simulink model "ScanMatcher_v21"  (R2021a)
settings: Solver=FixedStepAuto  StartTime=0.0  StopTime=inf  RelTol=1e-3
model workspace (MAT data in the model file):
  SL_ROS_VariableLengthArrays_MaxSizes.CommonInfo.ArrayTruncateAction = 'EmitWarning'
  SL_ROS_VariableLengthArrays_MaxSizes.MsgTypeMap = containers.Map
  SL_ROS_VariableLengthArrays_MaxSizes.MsgTypeMap.serialization.keys = {'sensor_msgs/LaserScan'}
  SL_ROS_VariableLengthArrays_MaxSizes.MsgTypeMap.serialization.values{1}(1).PropertyName = 'Intensities'
  SL_ROS_VariableLengthArrays_MaxSizes.MsgTypeMap.serialization.values{1}(1).DataType = 'single'
  SL_ROS_VariableLengthArrays_MaxSizes.MsgTypeMap.serialization.values{1}(1).MaxLength = 1084
  SL_ROS_VariableLengthArrays_MaxSizes.MsgTypeMap.serialization.values{1}(2).PropertyName = 'Ranges'
  SL_ROS_VariableLengthArrays_MaxSizes.MsgTypeMap.serialization.values{1}(2).DataType = 'single'
  SL_ROS_VariableLengthArrays_MaxSizes.MsgTypeMap.serialization.values{1}(2).MaxLength = 1084
  SL_ROS_VariableLengthArrays_MaxSizes.MsgTypeMap.serialization.uniformity = 0
  SL_ROS_VariableLengthArrays_MaxSizes.MsgTypeMap.serialization.keyType = 'char'
  SL_ROS_VariableLengthArrays_MaxSizes.MsgTypeMap.serialization.valueType = 'any'
undefined symbols (not defined in the file): Header, Pose, Theta, X, Y
libraries: robotlib x23, robotcorelib x2
(part 1 of 2)
settings Model: Creator=roboticlab01  LastModifiedBy=roboticlab02
settings SolverCC: AlgebraicLoopSolver=TrustRegion
settings OptimizationCC: EnhancedBackFolding=on  PassReuseOutputArgsAs=Individual arguments  MaxStackSize=64  OptimizeBlockOrder=speed  DifferentSizesBufferReuse=on  OptimizationCustomize=off  EfficientTunableParamExpr=on
settings DebuggingCC: ParameterTunabilityLossMsg=error  SFMachineParentedDataDiag=warning
settings HardwareCC: ProdBitPerPointer=32  ProdBitPerSizeT=32  ProdBitPerPtrDiffT=32  ProdLargestAtomicFloat=None  ProdIntDivRoundTo=Undefined  ProdEndianess=Unspecified  ProdWordSize=32  ProdHWDeviceType=Generic->Unspecified (assume 32-bit Generic)
settings SFSimCC: MATLABDynamicMemAlloc=off  CustomCodeUndefinedFunction=UseInterfaceOnly  SimTargetLang=C++
settings RTWCC: SystemTargetFile=ert.tlc  HardwareBoard=Robot Operating System (ROS)  TLCOptions="-aInlineSetEventsForThisBaseRateFcn=TLC_FALSE -aSuppressMultiTaskScheduler=TLC_FALSE  -aRateBasedStepFcn=0"  TemplateMakefile=ert_default_tmf  GenerateReport=on  Toolchain=Catkin  IncludeHyperlinkInReport=on  LaunchReport=on  TargetLang=C++  GenerateTraceInfo=on  GenerateTraceReport=on  GenerateTraceReportSl=on  GenerateTraceReportSf=on  GenerateTraceReportEml=on
settings CodeAppCC: ForceParamTrailComments=on  IgnoreCustomStorageClasses=off  OperatorAnnotations=on  SimulinkDataObjDesc=on  SFDataObjDesc=on  InsertBlockDesc=on
settings ERTTargetCC: SupportVariableSizeSignals=on

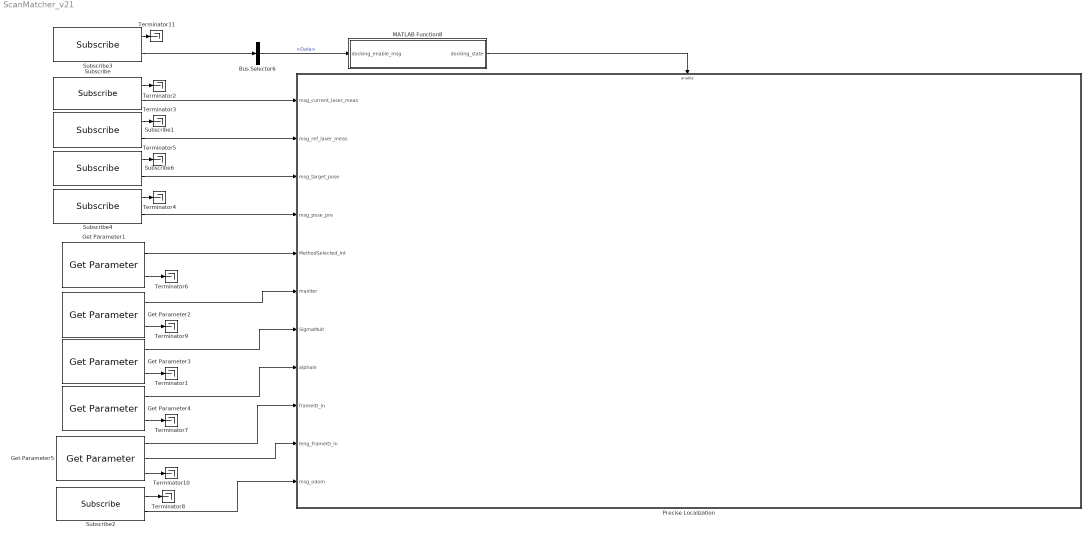
== system ScanMatcher_v21 ==
  Bus Selector6 : BusSelector  OutputSignals=Data
  Get Parameter1 : robotlib/Get Parameter  ParameterSource=Select from ROS network  ParameterName=/use_which_matcher  ParameterType=int32  ParameterMaxArrayLength=16  ParameterInitialValue=0  SampleTime=-1  ShowErrorCodeOutput=on  ModelName=ScanMatcher_v21  BlockId=ParamGet_ScanMatcher_v21_196
      settings: SourceProductBaseCode=RR
  Get Parameter2 : robotlib/Get Parameter  ParameterSource=Select from ROS network  ParameterName=/maxIter  ParameterType=int32  ParameterMaxArrayLength=16  ParameterInitialValue=100  SampleTime=-1  ShowErrorCodeOutput=on  ModelName=ScanMatcher_v21  BlockId=ParamGet_ScanMatcher_v21_325
      settings: SourceProductBaseCode=RR
  Get Parameter3 : robotlib/Get Parameter  ParameterSource=Select from ROS network  ParameterName=/sigmaMult  ParameterType=double  ParameterMaxArrayLength=16  ParameterInitialValue=1  SampleTime=-1  ShowErrorCodeOutput=on  ModelName=ScanMatcher_v21  BlockId=ParamGet_ScanMatcher_v21_340
      settings: SourceProductBaseCode=RR
  Get Parameter4 : robotlib/Get Parameter  ParameterSource=Select from ROS network  ParameterName=/alphaIn  ParameterType=double  ParameterMaxArrayLength=16  ParameterInitialValue=0.8  SampleTime=-1  ShowErrorCodeOutput=on  ModelName=ScanMatcher_v21  BlockId=ParamGet_ScanMatcher_v21_351
      settings: SourceProductBaseCode=RR
  Get Parameter5 : robotlib/Get Parameter  ParameterSource=Select from ROS network  ParameterName=/pose_frameID  ParameterType=uint8[] (string)  ParameterMaxArrayLength=32  ParameterInitialValue=0  SampleTime=-1  ShowErrorCodeOutput=on  ModelName=ScanMatcher_v21  BlockId=ParamGet_ScanMatcher_v21_466
      settings: SourceProductBaseCode=RR
  MATLAB Function8 : MATLAB Function  TreatAsAtomicUnit=on
  Precise Localization : Subsystem
  Subscribe : robotlib/Subscribe  topicSource=Select from ROS network  topic=/laser_all  messageType=sensor_msgs/LaserScan  SampleTime=-1  legacyBusStruct=off  messageQueueLength=1
  Subscribe1 : robotlib/Subscribe  topicSource=Specify your own  topic=/laser_all_ref  messageType=sensor_msgs/LaserScan  SampleTime=-1  legacyBusStruct=off  messageQueueLength=1
  Subscribe2 : robotlib/Subscribe  topicSource=Select from ROS network  topic=/odom  messageType=nav_msgs/Odometry  SampleTime=-1  legacyBusStruct=off  messageQueueLength=1
  Subscribe3 : robotlib/Subscribe  topicSource=Select from ROS network  topic=/enable_docking  messageType=std_msgs/Bool  SampleTime=-1  legacyBusStruct=off  messageQueueLength=2
      settings: SourceProductBaseCode=RO
  Subscribe4 : robotlib/Subscribe  topicSource=Specify your own  topic=/pose_estim_pre  messageType=geometry_msgs/PoseWithCovarianceStamped  SampleTime=-1  legacyBusStruct=off  messageQueueLength=1
      settings: SourceProductBaseCode=RO
  Subscribe6 : robotlib/Subscribe  topicSource=Select from ROS network  topic=/target_pose  messageType=geometry_msgs/Pose2D  SampleTime=-1  legacyBusStruct=off  messageQueueLength=1
      settings: SourceProductBaseCode=RO
  Terminator{1..11} (11 alike) : Terminator
  wires:
  Subscribe/1 -> Terminator2/1
  Subscribe1/1 -> Terminator3/1
  Subscribe4/1 -> Terminator4/1
  Subscribe6/1 -> Terminator5/1
  Get Parameter1/2 -> Terminator6/1
  Get Parameter2/2 -> Terminator9/1
  Get Parameter3/2 -> Terminator1/1
  Get Parameter4/2 -> Terminator7/1
  Subscribe2/1 -> Terminator8/1
  Get Parameter5/3 -> Terminator10/1
  Subscribe/2 -> Precise Localization/1(msg_current_laser_meas)
  Subscribe1/2 -> Precise Localization/2(msg_ref_laser_meas)
  Subscribe6/2 -> Precise Localization/3(msg_target_pose)
  Subscribe4/2 -> Precise Localization/4(msg_pose_pre)
  Get Parameter1/1 -> Precise Localization/5(MethodSelected_Int)
  Get Parameter2/1 -> Precise Localization/6(maxIter)
  Get Parameter3/1 -> Precise Localization/7(SigmaMult)
  Get Parameter4/1 -> Precise Localization/8(alphaIn)
  Get Parameter5/1 -> Precise Localization/9(frameID_in)
  Get Parameter5/2 -> Precise Localization/10(leng_frameID_in)
  Subscribe2/2 -> Precise Localization/11(msg_odom)
  Subscribe3/1 -> Terminator11/1
  MATLAB Function8/1(docking_state) -> Precise Localization/Enable
  Subscribe3/2 -> Bus Selector6/1
  Bus Selector6/1 -> MATLAB Function8/1(docking_enable_msg)  "<Data>"

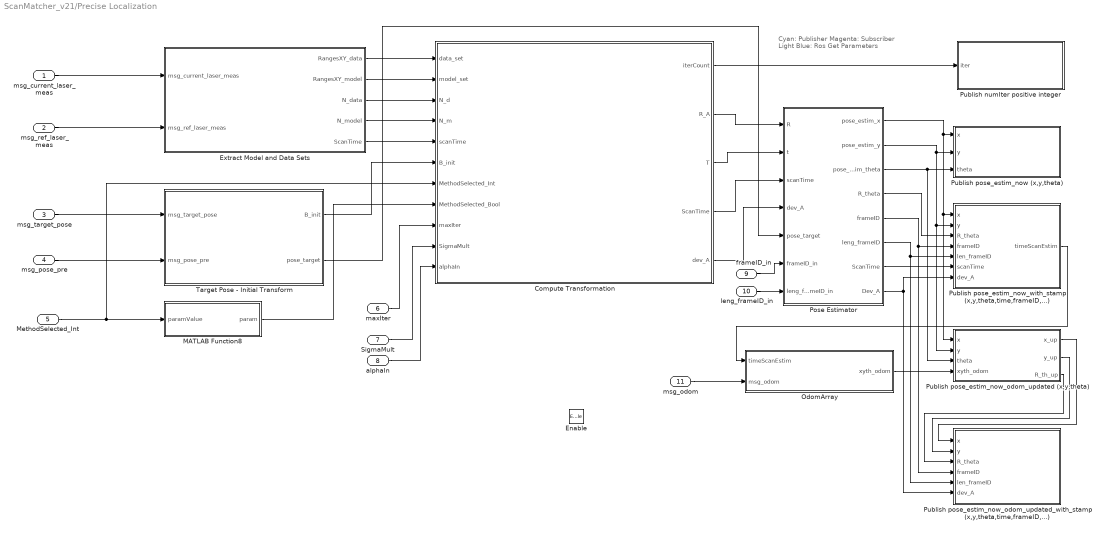
== system ScanMatcher_v21/Precise Localization ==
  note: Cyan: Publisher
      | Magenta: Subscriber
      | Light Blue: Ros Get Parameters
  msg_current_laser_meas : Inport
  msg_ref_laser_meas : Inport  Port=2
  msg_target_pose : Inport  Port=3
  msg_pose_pre : Inport  Port=4
  MethodSelected_Int : Inport  Port=5
  maxIter : Inport  Port=6
  SigmaMult : Inport  Port=7
  alphaIn : Inport  Port=8
  frameID_in : Inport  Port=9
  leng_frameID_in : Inport  Port=10
  msg_odom : Inport  Port=11
  Enable : EnablePort  PropagateVarSize=During execution
  Compute Transformation : Subsystem
  Extract Model and Data Sets : Subsystem
  MATLAB Function8 : MATLAB Function  TreatAsAtomicUnit=on
  OdomArray : Subsystem
  Pose Estimator : MATLAB Function  TreatAsAtomicUnit=on
  Publish numIter positive integer : Subsystem
  Publish pose_estim_now (x,y,theta) : Subsystem
  Publish pose_estim_now_odom_updated (x,y,theta) : Subsystem
  Publish pose_estim_now_odom_updated_with_stamp (x,y,theta,time,frameID,...) : Subsystem
  Publish pose_estim_now_with_stamp (x,y,theta,time,frameID,...) : Subsystem
  Target Pose - Initial Transform : Subsystem
  wires:
  Compute Transformation/1(iterCount) -> Publish numIter positive integer/1(iter)
  Publish pose_estim_now_odom_updated (x,y,theta)/1(x_up) -> Publish pose_estim_now_odom_updated_with_stamp (x,y,theta,time,frameID,...)/1(x)
  Extract Model and Data Sets/5(ScanTime) -> Compute Transformation/5(scanTime)
  msg_pose_pre/1 -> Target Pose - Initial Transform/2(msg_pose_pre)
  Pose Estimator/8(Dev_A) -> Publish pose_estim_now_with_stamp (x,y,theta,time,frameID,...)/7(dev_A), Publish pose_estim_now_odom_updated_with_stamp (x,y,theta,time,frameID,...)/6(dev_A)
  Compute Transformation/4(ScanTime) -> Pose Estimator/3(scanTime)
  msg_ref_laser_meas/1 -> Extract Model and Data Sets/2(msg_ref_laser_meas)
  MethodSelected_Int/1 -> Compute Transformation/7(MethodSelected_Int), MATLAB Function8/1(paramValue)
  alphaIn/1 -> Compute Transformation/11(alphaIn)
  Compute Transformation/2(R_A) -> Pose Estimator/1(R)
  maxIter/1 -> Compute Transformation/9(maxIter)
  Pose Estimator/3(pose_estim_theta) -> Publish pose_estim_now (x,y,theta)/3(theta), Publish pose_estim_now_odom_updated (x,y,theta)/3(theta)
  Compute Transformation/3(T) -> Pose Estimator/2(t)
  leng_frameID_in/1 -> Pose Estimator/7(leng_frameID_in)
  MATLAB Function8/1(param) -> Compute Transformation/8(MethodSelected_Bool)
  msg_target_pose/1 -> Target Pose - Initial Transform/1(msg_target_pose)
  Pose Estimator/5(frameID) -> Publish pose_estim_now_odom_updated_with_stamp (x,y,theta,time,frameID,...)/4(frameID), Publish pose_estim_now_with_stamp (x,y,theta,time,frameID,...)/4(frameID)
  Extract Model and Data Sets/2(RangesXY_model) -> Compute Transformation/2(model_set)
  SigmaMult/1 -> Compute Transformation/10(SigmaMult)
  msg_current_laser_meas/1 -> Extract Model and Data Sets/1(msg_current_laser_meas)
  Compute Transformation/5(dev_A) -> Pose Estimator/4(dev_A)
  Target Pose - Initial Transform/1(B_init) -> Compute Transformation/6(B_init)
  Pose Estimator/2(pose_estim_y) -> Publish pose_estim_now_odom_updated (x,y,theta)/2(y), Publish pose_estim_now_with_stamp (x,y,theta,time,frameID,...)/2(y), Publish pose_estim_now (x,y,theta)/2(y)
  Pose Estimator/6(leng_frameID) -> Publish pose_estim_now_odom_updated_with_stamp (x,y,theta,time,frameID,...)/5(len_frameID), Publish pose_estim_now_with_stamp (x,y,theta,time,frameID,...)/5(len_frameID)
  Pose Estimator/1(pose_estim_x) -> Publish pose_estim_now_odom_updated (x,y,theta)/1(x), Publish pose_estim_now_with_stamp (x,y,theta,time,frameID,...)/1(x), Publish pose_estim_now (x,y,theta)/1(x)
  Publish pose_estim_now_odom_updated (x,y,theta)/3(R_th_up) -> Publish pose_estim_now_odom_updated_with_stamp (x,y,theta,time,frameID,...)/3(R_theta)
  Target Pose - Initial Transform/2(pose_target) -> Pose Estimator/5(pose_target)
  Pose Estimator/4(R_theta) -> Publish pose_estim_now_with_stamp (x,y,theta,time,frameID,...)/3(R_theta)
  frameID_in/1 -> Pose Estimator/6(frameID_in)
  Extract Model and Data Sets/1(RangesXY_data) -> Compute Transformation/1(data_set)
  Extract Model and Data Sets/3(N_data) -> Compute Transformation/3(N_d)
  Pose Estimator/7(ScanTime) -> Publish pose_estim_now_with_stamp (x,y,theta,time,frameID,...)/6(scanTime)
  OdomArray/1(xyth_odom) -> Publish pose_estim_now_odom_updated (x,y,theta)/4(xyth_odom)
  Publish pose_estim_now_odom_updated (x,y,theta)/2(y_up) -> Publish pose_estim_now_odom_updated_with_stamp (x,y,theta,time,frameID,...)/2(y)
  Extract Model and Data Sets/4(N_model) -> Compute Transformation/4(N_m)
  msg_odom/1 -> OdomArray/2(msg_odom)
  Publish pose_estim_now_with_stamp (x,y,theta,time,frameID,...)/1(timeScanEstim) -> OdomArray/1(timeScanEstim)

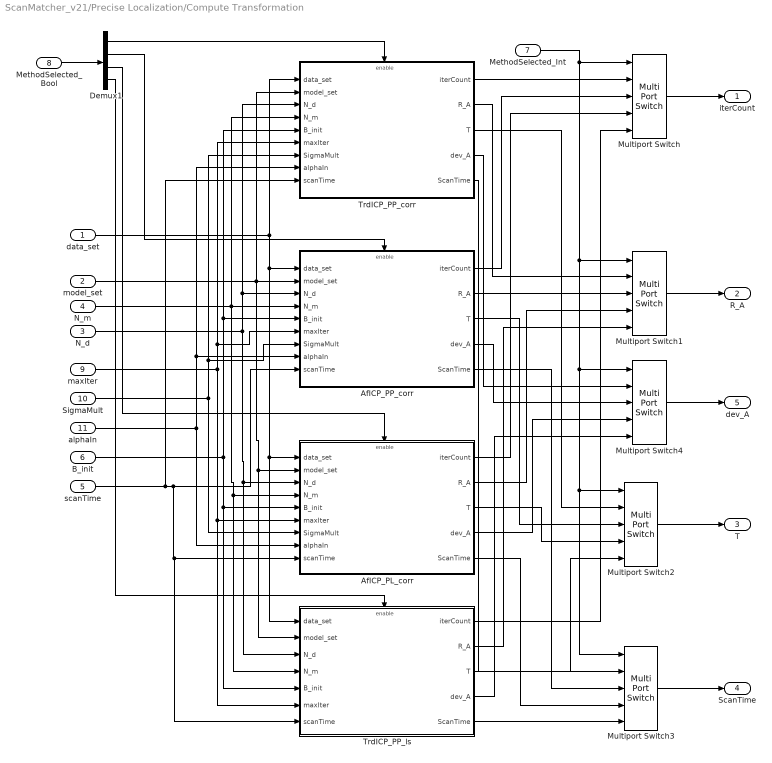
== system ScanMatcher_v21/Precise Localization/Compute Transformation ==
  data_set : Inport
  model_set : Inport  Port=2
  N_d : Inport  Port=3
  N_m : Inport  Port=4
  scanTime : Inport  Port=5
  B_init : Inport  Port=6
  MethodSelected_Int : Inport  Port=7
  MethodSelected_Bool : Inport  Port=8
  maxIter : Inport  Port=9
  SigmaMult : Inport  Port=10
  alphaIn : Inport  Port=11
  AfICP_PL_corr : Subsystem  TreatAsAtomicUnit=on
  AfICP_PP_corr : Subsystem  TreatAsAtomicUnit=on
  Demux1 : Demux
  Multiport Switch{,1..4} (5 alike) : MultiPortSwitch  Inputs=4
  TrdICP_PP_corr : Subsystem  TreatAsAtomicUnit=on
  TrdICP_PP_ls : Subsystem  TreatAsAtomicUnit=on
  iterCount : Outport
  R_A : Outport  Port=2
  T : Outport  Port=3
  ScanTime : Outport  Port=4
  dev_A : Outport  Port=5
  wires:
  AfICP_PL_corr/2(R_A) -> Multiport Switch1/4
  AfICP_PP_corr/2(R_A) -> Multiport Switch1/3
  TrdICP_PP_corr/2(R_A) -> Multiport Switch1/2
  data_set/1 -> TrdICP_PP_ls/1(data_set), AfICP_PL_corr/1(data_set), AfICP_PP_corr/1(data_set), TrdICP_PP_corr/1(data_set)
  AfICP_PL_corr/1(iterCount) -> Multiport Switch/4
  TrdICP_PP_ls/2(R_A) -> Multiport Switch1/5
  TrdICP_PP_corr/3(T) -> Multiport Switch2/2
  TrdICP_PP_ls/3(T) -> Multiport Switch2/5
  Demux1/4 -> TrdICP_PP_ls/Enable
  B_init/1 -> TrdICP_PP_corr/5(B_init), AfICP_PP_corr/5(B_init), TrdICP_PP_ls/5(B_init), AfICP_PL_corr/5(B_init)
  model_set/1 -> TrdICP_PP_corr/2(model_set), AfICP_PP_corr/2(model_set), TrdICP_PP_ls/2(model_set), AfICP_PL_corr/2(model_set)
  AfICP_PP_corr/1(iterCount) -> Multiport Switch/3
  Demux1/3 -> AfICP_PL_corr/Enable
  N_m/1 -> TrdICP_PP_ls/4(N_m), AfICP_PL_corr/4(N_m), AfICP_PP_corr/4(N_m), TrdICP_PP_corr/4(N_m)
  maxIter/1 -> TrdICP_PP_corr/6(maxIter), AfICP_PP_corr/6(maxIter), TrdICP_PP_ls/6(maxIter), AfICP_PL_corr/6(maxIter)
  Demux1/2 -> AfICP_PP_corr/Enable
  Demux1/1 -> TrdICP_PP_corr/Enable
  MethodSelected_Bool/1 -> Demux1/1
  TrdICP_PP_corr/1(iterCount) -> Multiport Switch/2
  AfICP_PL_corr/3(T) -> Multiport Switch2/4
  AfICP_PP_corr/3(T) -> Multiport Switch2/3
  TrdICP_PP_ls/1(iterCount) -> Multiport Switch/5
  N_d/1 -> TrdICP_PP_corr/3(N_d), AfICP_PP_corr/3(N_d), TrdICP_PP_ls/3(N_d), AfICP_PL_corr/3(N_d)
  Multiport Switch/1 -> iterCount/1
  Multiport Switch1/1 -> R_A/1
  Multiport Switch2/1 -> T/1
  MethodSelected_Int/1 -> Multiport Switch4/1, Multiport Switch3/1, Multiport Switch2/1, Multiport Switch1/1, Multiport Switch/1
  SigmaMult/1 -> AfICP_PL_corr/7(SigmaMult), TrdICP_PP_corr/7(SigmaMult), AfICP_PP_corr/7(SigmaMult)
  alphaIn/1 -> TrdICP_PP_corr/8(alphaIn), AfICP_PP_corr/8(alphaIn), AfICP_PL_corr/8(alphaIn)
  scanTime/1 -> TrdICP_PP_corr/9(scanTime), TrdICP_PP_ls/7(scanTime), AfICP_PL_corr/9(scanTime), AfICP_PP_corr/9(scanTime)
  Multiport Switch3/1 -> ScanTime/1
  TrdICP_PP_corr/5(ScanTime) -> Multiport Switch3/2
  AfICP_PP_corr/5(ScanTime) -> Multiport Switch3/3
  AfICP_PL_corr/5(ScanTime) -> Multiport Switch3/4
  TrdICP_PP_ls/5(ScanTime) -> Multiport Switch3/5
  Multiport Switch4/1 -> dev_A/1
  AfICP_PP_corr/4(dev_A) -> Multiport Switch4/3
  AfICP_PL_corr/4(dev_A) -> Multiport Switch4/4
  TrdICP_PP_corr/4(dev_A) -> Multiport Switch4/2
  TrdICP_PP_ls/4(dev_A) -> Multiport Switch4/5

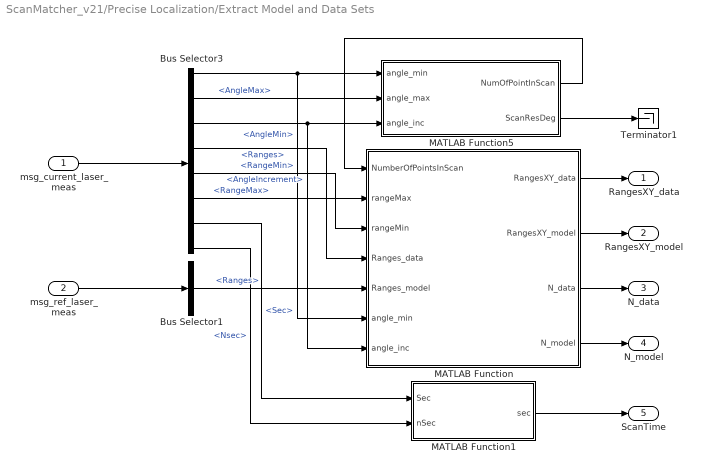
== system ScanMatcher_v21/Precise Localization/Extract Model and Data Sets ==
  msg_current_laser_meas : Inport
  msg_ref_laser_meas : Inport  Port=2
  Bus Selector1 : BusSelector  OutputSignals=Ranges
  Bus Selector3 : BusSelector  OutputSignals=AngleMin,AngleMax,AngleIncrement,Ranges,RangeMin,RangeMax,Header.Stamp.Sec,Header.Stamp.Nsec
  MATLAB Function : MATLAB Function  TreatAsAtomicUnit=on
  MATLAB Function1 : MATLAB Function  TreatAsAtomicUnit=on
  MATLAB Function5 : MATLAB Function  TreatAsAtomicUnit=on
  Terminator1 : Terminator
  RangesXY_data : Outport
  RangesXY_model : Outport  Port=2
  N_data : Outport  Port=3
  N_model : Outport  Port=4
  ScanTime : Outport  Port=5
  wires:
  MATLAB Function/1(RangesXY_data) -> RangesXY_data/1
  Bus Selector3/6 -> MATLAB Function/2(rangeMax)  "<RangeMax>"
  MATLAB Function5/1(NumOfPointInScan) -> MATLAB Function/1(NumberOfPointsInScan)
  Bus Selector3/1 -> MATLAB Function/6(angle_min), MATLAB Function5/1(angle_min)  "<AngleMin>"
  msg_current_laser_meas/1 -> Bus Selector3/1
  MATLAB Function/2(RangesXY_model) -> RangesXY_model/1
  MATLAB Function/3(N_data) -> N_data/1
  Bus Selector3/4 -> MATLAB Function/4(Ranges_data)  "<Ranges>"
  msg_ref_laser_meas/1 -> Bus Selector1/1
  MATLAB Function/4(N_model) -> N_model/1
  Bus Selector3/5 -> MATLAB Function/3(rangeMin)  "<RangeMin>"
  Bus Selector3/3 -> MATLAB Function/7(angle_inc), MATLAB Function5/3(angle_inc)  "<AngleIncrement>"
  Bus Selector3/2 -> MATLAB Function5/2(angle_max)  "<AngleMax>"
  Bus Selector1/1 -> MATLAB Function/5(Ranges_model)  "<Ranges>"
  MATLAB Function5/2(ScanResDeg) -> Terminator1/1
  Bus Selector3/7 -> MATLAB Function1/1(Sec)  "<Sec>"
  Bus Selector3/8 -> MATLAB Function1/2(nSec)  "<Nsec>"
  MATLAB Function1/1(sec) -> ScanTime/1

== system ScanMatcher_v21/Precise Localization/OdomArray ==
  timeScanEstim : Inport
  msg_odom : Inport  Port=2
  Bus Selector1 : BusSelector  OutputSignals=Pose.Pose.Position.X,Pose.Pose.Position.Y,Pose.Pose.Orientation.W,Pose.Pose.Orientation.X,Pose.Pose.Orientation.Y,Pose.Pose.Orientation.Z
  Bus Selector6 : BusSelector  OutputSignals=Header.Stamp.Sec,Header.Stamp.Nsec,Twist.Twist.Linear.X,Twist.Twist.Angular.Z
  MATLAB Function2 : MATLAB Function  TreatAsAtomicUnit=on
  MATLAB Function3 : MATLAB Function  TreatAsAtomicUnit=on
  MATLAB Function5 : MATLAB Function  TreatAsAtomicUnit=on
  Memory4 : Memory  InitialCondition=zeros(50,6)
  Mux2 : Mux
  xyth_odom : Outport
  wires:
  Bus Selector1/6 -> Mux2/4  "<Z>"
  MATLAB Function2/1(theta) -> MATLAB Function5/3(pos_th)
  Mux2/1 -> MATLAB Function2/1(quat_In)
  Bus Selector1/3 -> Mux2/1  "<W>"
  Bus Selector1/2 -> MATLAB Function5/2(pos_y)  "<Y>"
  MATLAB Function5/1(ArrayOdomNow) -> Memory4/1, MATLAB Function3/2(OdomArray)
  Bus Selector1/1 -> MATLAB Function5/1(pos_x)  "<X>"
  Bus Selector1/5 -> Mux2/3  "<Y>"
  Bus Selector1/4 -> Mux2/2  "<X>"
  Bus Selector6/4 -> MATLAB Function5/7(vel_w_z)  "<Z>"
  msg_odom/1 -> Bus Selector6/1, Bus Selector1/1
  Bus Selector6/1 -> MATLAB Function5/4(Sec)  "<Sec>"
  Bus Selector6/3 -> MATLAB Function5/6(vel_x)  "<X>"
  Memory4/1 -> MATLAB Function5/8(ArrayOdomLast)
  Bus Selector6/2 -> MATLAB Function5/5(nSec)  "<Nsec>"
  timeScanEstim/1 -> MATLAB Function3/1(ScanEstimTime)
  MATLAB Function3/1(xyth_odom) -> xyth_odom/1

== system ScanMatcher_v21/Precise Localization/Publish numIter positive integer ==
  iter : Inport
  Blank Message2 : robotlib/Blank Message  messageClass=Message  entityType=std_msgs/Int16  messageType=std_msgs/Int16  SampleTime=inf  legacyBusStruct=off
      settings: SourceProductBaseCode=RO
  Bus Assignment2 : BusAssignment  AssignedSignals=Data
  Publish1 : robotlib/Publish  topicSource=Specify your own  topic=/numIter  messageType=std_msgs/Int16  legacyBusStruct=off  messageQueueLength=1
      settings: SourceProductBaseCode=RO
  wires:
  Bus Assignment2/1 -> Publish1/1
  iter/1 -> Bus Assignment2/2
  Blank Message2/1 -> Bus Assignment2/1

== system ScanMatcher_v21/Precise Localization/Publish pose_estim_now (x,y,theta) ==
  x : Inport
  y : Inport  Port=2
  theta : Inport  Port=3
  Blank Message1 : robotlib/Blank Message  messageClass=Message  entityType=geometry_msgs/Pose2D  messageType=geometry_msgs/Pose2D  SampleTime=inf  legacyBusStruct=off
      settings: SourceProductBaseCode=RO
  Bus Assignment1 : BusAssignment  AssignedSignals=X,Y,Theta
  Publish : robotlib/Publish  topicSource=Specify your own  topic=/pose_estim_now  messageType=geometry_msgs/Pose2D  legacyBusStruct=off  messageQueueLength=1
      settings: SourceProductBaseCode=RO
  wires:
  Blank Message1/1 -> Bus Assignment1/1
  Bus Assignment1/1 -> Publish/1
  y/1 -> Bus Assignment1/3
  theta/1 -> Bus Assignment1/4
  x/1 -> Bus Assignment1/2

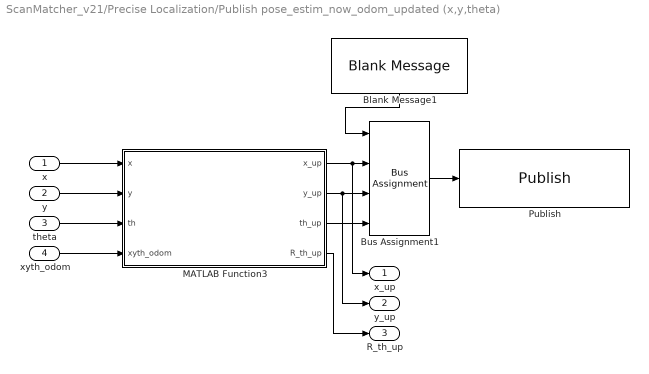
== system ScanMatcher_v21/Precise Localization/Publish pose_estim_now_odom_updated (x,y,theta) ==
  x : Inport
  y : Inport  Port=2
  theta : Inport  Port=3
  xyth_odom : Inport  Port=4
  Blank Message1 : robotlib/Blank Message  messageClass=Message  entityType=geometry_msgs/Pose2D  messageType=geometry_msgs/Pose2D  SampleTime=inf  legacyBusStruct=off
      settings: SourceProductBaseCode=RO
  Bus Assignment1 : BusAssignment  AssignedSignals=X,Y,Theta
  MATLAB Function3 : MATLAB Function  TreatAsAtomicUnit=on
  Publish : robotlib/Publish  topicSource=Specify your own  topic=/pose_estim_now_odom_upd  messageType=geometry_msgs/Pose2D  legacyBusStruct=off  messageQueueLength=1
      settings: SourceProductBaseCode=RO
  x_up : Outport
  y_up : Outport  Port=2
  R_th_up : Outport  Port=3
  wires:
  Blank Message1/1 -> Bus Assignment1/1
  Bus Assignment1/1 -> Publish/1
  MATLAB Function3/1(x_up) -> x_up/1, Bus Assignment1/2
  MATLAB Function3/2(y_up) -> Bus Assignment1/3, y_up/1
  MATLAB Function3/3(th_up) -> Bus Assignment1/4
  x/1 -> MATLAB Function3/1(x)
  y/1 -> MATLAB Function3/2(y)
  theta/1 -> MATLAB Function3/3(th)
  xyth_odom/1 -> MATLAB Function3/4(xyth_odom)
  MATLAB Function3/4(R_th_up) -> R_th_up/1

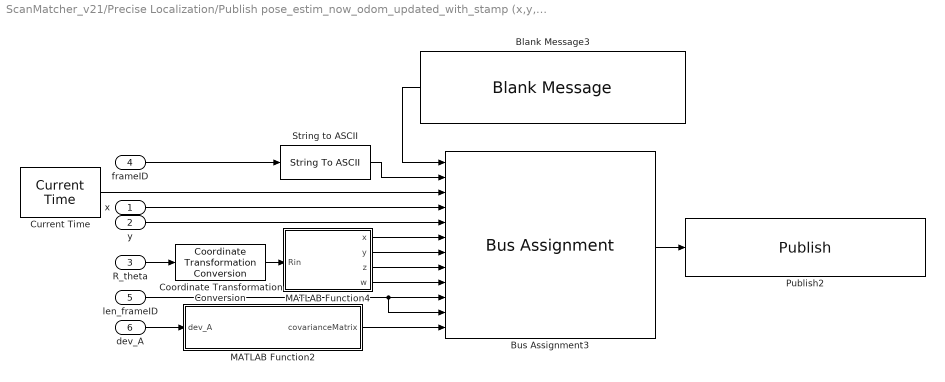
== system ScanMatcher_v21/Precise Localization/Publish pose_estim_now_odom_updated_with_stamp (x,y,theta,time,frameID,...) ==
  x : Inport
  y : Inport  Port=2
  R_theta : Inport  Port=3
  frameID : Inport  Port=4
  len_frameID : Inport  Port=5
  dev_A : Inport  Port=6
  Blank Message3 : robotlib/Blank Message  messageClass=Message  entityType=geometry_msgs/PoseWithCovarianceStamped  messageType=geometry_msgs/PoseWithCovarianceStamped  SampleTime=inf  legacyBusStruct=off
      settings: SourceProductBaseCode=RO
  Bus Assignment3 : BusAssignment  AssignedSignals=Header.FrameId,Header.Stamp,Pose.Pose.Position.X,Pose.Pose.Position.Y,Pose.Pose.Orientation.X,Pose.Pose.Orientation.Y,Pose.Pose.Orientation.Z,Pose.Pose.Orientation.W,Header.FrameId_SL_Info.CurrentLength,Header.FrameId_SL_Info.ReceivedLength,Pose.Covariance
  Coordinate Transformation Conversion : robotcorelib/Coordinate Transformation Conversion  InputRepresentation=Rotation Matrix  InputEulerSequence=ZYX  ShowTrVecInputPort=on  OutputRepresentation=Quaternion  OutputEulerSequence=ZYX  ShowTrVecOutputPort=on  SimulateUsing=Code generation
      settings: SourceProductBaseCode=RO
  Current Time : robotlib/Current Time  OutputFormat=bus  SampleTime=-1  ModelName=ScanMatcher_v21
      settings: SourceProductBaseCode=RR
  MATLAB Function2 : MATLAB Function  TreatAsAtomicUnit=on
  MATLAB Function4 : MATLAB Function  TreatAsAtomicUnit=on
  Publish2 : robotlib/Publish  topicSource=Specify your own  topic=/pose_estim_now_odom_upd_with_stamp  messageType=geometry_msgs/PoseWithCovarianceStamped  legacyBusStruct=off  messageQueueLength=1
      settings: SourceProductBaseCode=RO
  String to ASCII : StringToASCII  OutputVectorSize=128
  wires:
  Bus Assignment3/1 -> Publish2/1
  Coordinate Transformation Conversion/1 -> MATLAB Function4/1(Rin)
  len_frameID/1 -> Bus Assignment3/11, Bus Assignment3/10
  Current Time/1 -> Bus Assignment3/3
  MATLAB Function4/1(x) -> Bus Assignment3/6
  MATLAB Function4/4(w) -> Bus Assignment3/9
  y/1 -> Bus Assignment3/5
  String to ASCII/1 -> Bus Assignment3/2
  frameID/1 -> String to ASCII/1
  Blank Message3/1 -> Bus Assignment3/1
  x/1 -> Bus Assignment3/4
  R_theta/1 -> Coordinate Transformation Conversion/1
  MATLAB Function4/3(z) -> Bus Assignment3/8
  MATLAB Function4/2(y) -> Bus Assignment3/7
  dev_A/1 -> MATLAB Function2/1(dev_A)
  MATLAB Function2/1(covarianceMatrix) -> Bus Assignment3/12

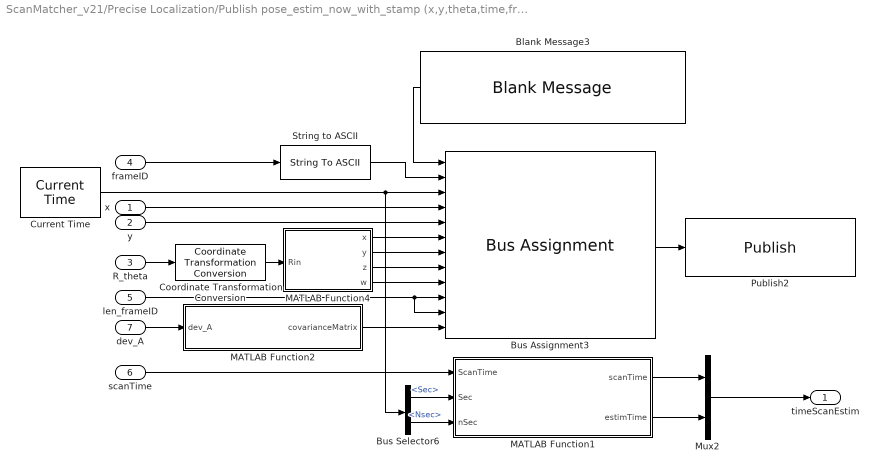
== system ScanMatcher_v21/Precise Localization/Publish pose_estim_now_with_stamp (x,y,theta,time,frameID,...) ==
  x : Inport
  y : Inport  Port=2
  R_theta : Inport  Port=3
  frameID : Inport  Port=4
  len_frameID : Inport  Port=5
  scanTime : Inport  Port=6
  dev_A : Inport  Port=7
  Blank Message3 : robotlib/Blank Message  messageClass=Message  entityType=geometry_msgs/PoseWithCovarianceStamped  messageType=geometry_msgs/PoseWithCovarianceStamped  SampleTime=inf  legacyBusStruct=off
      settings: SourceProductBaseCode=RO
  Bus Assignment3 : BusAssignment  AssignedSignals=Header.FrameId,Header.Stamp,Pose.Pose.Position.X,Pose.Pose.Position.Y,Pose.Pose.Orientation.X,Pose.Pose.Orientation.Y,Pose.Pose.Orientation.Z,Pose.Pose.Orientation.W,Header.FrameId_SL_Info.CurrentLength,Header.FrameId_SL_Info.ReceivedLength,Pose.Covariance
  Bus Selector6 : BusSelector  OutputSignals=Sec,Nsec
  Coordinate Transformation Conversion : robotcorelib/Coordinate Transformation Conversion  InputRepresentation=Rotation Matrix  InputEulerSequence=ZYX  ShowTrVecInputPort=on  OutputRepresentation=Quaternion  OutputEulerSequence=ZYX  ShowTrVecOutputPort=on  SimulateUsing=Code generation
      settings: SourceProductBaseCode=RO
  Current Time : robotlib/Current Time  OutputFormat=bus  SampleTime=-1  ModelName=ScanMatcher_v21
      settings: SourceProductBaseCode=RR
  MATLAB Function1 : MATLAB Function  TreatAsAtomicUnit=on
  MATLAB Function2 : MATLAB Function  TreatAsAtomicUnit=on
  MATLAB Function4 : MATLAB Function  TreatAsAtomicUnit=on
  Mux2 : Mux  Inputs=2
  Publish2 : robotlib/Publish  topicSource=Specify your own  topic=/pose_estim_now_with_stamp  messageType=geometry_msgs/PoseWithCovarianceStamped  legacyBusStruct=off  messageQueueLength=1
      settings: SourceProductBaseCode=RO
  String to ASCII : StringToASCII  OutputVectorSize=128
  timeScanEstim : Outport
  wires:
  Bus Assignment3/1 -> Publish2/1
  Coordinate Transformation Conversion/1 -> MATLAB Function4/1(Rin)
  len_frameID/1 -> Bus Assignment3/11, Bus Assignment3/10
  Current Time/1 -> Bus Selector6/1, Bus Assignment3/3
  MATLAB Function4/1(x) -> Bus Assignment3/6
  MATLAB Function4/4(w) -> Bus Assignment3/9
  y/1 -> Bus Assignment3/5
  String to ASCII/1 -> Bus Assignment3/2
  frameID/1 -> String to ASCII/1
  Blank Message3/1 -> Bus Assignment3/1
  x/1 -> Bus Assignment3/4
  R_theta/1 -> Coordinate Transformation Conversion/1
  MATLAB Function4/3(z) -> Bus Assignment3/8
  MATLAB Function4/2(y) -> Bus Assignment3/7
  scanTime/1 -> MATLAB Function1/1(ScanTime)
  Bus Selector6/1 -> MATLAB Function1/2(Sec)  "<Sec>"
  Bus Selector6/2 -> MATLAB Function1/3(nSec)  "<Nsec>"
  MATLAB Function1/1(scanTime) -> Mux2/1
  MATLAB Function1/2(estimTime) -> Mux2/2
  Mux2/1 -> timeScanEstim/1
  MATLAB Function2/1(covarianceMatrix) -> Bus Assignment3/12
  dev_A/1 -> MATLAB Function2/1(dev_A)

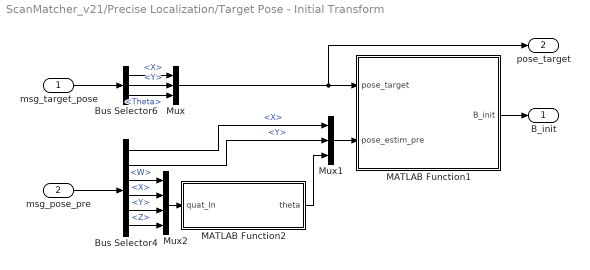
== system ScanMatcher_v21/Precise Localization/Target Pose - Initial Transform ==
  msg_target_pose : Inport
  msg_pose_pre : Inport  Port=2
  Bus Selector4 : BusSelector  OutputSignals=Pose.Pose.Position.X,Pose.Pose.Position.Y,Pose.Pose.Orientation.W,Pose.Pose.Orientation.X,Pose.Pose.Orientation.Y,Pose.Pose.Orientation.Z
  Bus Selector6 : BusSelector  OutputSignals=X,Y,Theta
  MATLAB Function1 : MATLAB Function  TreatAsAtomicUnit=on
  MATLAB Function2 : MATLAB Function  TreatAsAtomicUnit=on
  Mux : Mux  Inputs=3
  Mux1 : Mux  Inputs=3
  Mux2 : Mux
  B_init : Outport
  pose_target : Outport  Port=2
  wires:
  Bus Selector6/2 -> Mux/2  "<Y>"
  Bus Selector4/3 -> Mux2/1  "<W>"
  Bus Selector4/4 -> Mux2/2  "<X>"
  Mux2/1 -> MATLAB Function2/1(quat_In)
  Bus Selector4/2 -> Mux1/2  "<Y>"
  Bus Selector4/6 -> Mux2/4  "<Z>"
  MATLAB Function2/1(theta) -> Mux1/3
  msg_pose_pre/1 -> Bus Selector4/1
  Bus Selector4/1 -> Mux1/1  "<X>"
  Bus Selector4/5 -> Mux2/3  "<Y>"
  MATLAB Function1/1(B_init) -> B_init/1
  Bus Selector6/3 -> Mux/3  "<Theta>"
  msg_target_pose/1 -> Bus Selector6/1
  Bus Selector6/1 -> Mux/1  "<X>"
  Mux/1 -> pose_target/1, MATLAB Function1/1(pose_target)
  Mux1/1 -> MATLAB Function1/2(pose_estim_pre)

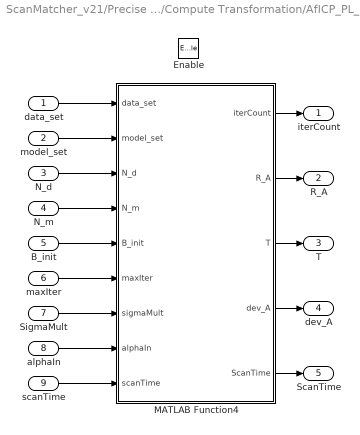
== system ScanMatcher_v21/Precise Localization/Compute Transformation/AfICP_PL_corr ==
  data_set : Inport
  model_set : Inport  Port=2
  N_d : Inport  Port=3
  N_m : Inport  Port=4
  B_init : Inport  Port=5
  maxIter : Inport  Port=6
  SigmaMult : Inport  Port=7
  alphaIn : Inport  Port=8
  scanTime : Inport  Port=9
  Enable : EnablePort
  MATLAB Function4 : MATLAB Function  TreatAsAtomicUnit=on
  iterCount : Outport
  R_A : Outport  Port=2
  T : Outport  Port=3
  dev_A : Outport  Port=4
  ScanTime : Outport  Port=5
  wires:
  data_set/1 -> MATLAB Function4/1(data_set)
  model_set/1 -> MATLAB Function4/2(model_set)
  N_d/1 -> MATLAB Function4/3(N_d)
  N_m/1 -> MATLAB Function4/4(N_m)
  B_init/1 -> MATLAB Function4/5(B_init)
  maxIter/1 -> MATLAB Function4/6(maxIter)
  MATLAB Function4/1(iterCount) -> iterCount/1
  MATLAB Function4/2(R_A) -> R_A/1
  MATLAB Function4/3(T) -> T/1
  SigmaMult/1 -> MATLAB Function4/7(sigmaMult)
  alphaIn/1 -> MATLAB Function4/8(alphaIn)
  scanTime/1 -> MATLAB Function4/9(scanTime)
  MATLAB Function4/5(ScanTime) -> ScanTime/1
  MATLAB Function4/4(dev_A) -> dev_A/1

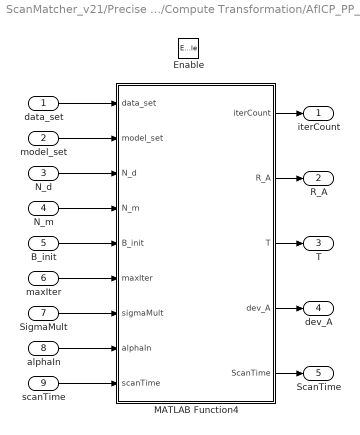
== system ScanMatcher_v21/Precise Localization/Compute Transformation/AfICP_PP_corr ==
  data_set : Inport
  model_set : Inport  Port=2
  N_d : Inport  Port=3
  N_m : Inport  Port=4
  B_init : Inport  Port=5
  maxIter : Inport  Port=6
  SigmaMult : Inport  Port=7
  alphaIn : Inport  Port=8
  scanTime : Inport  Port=9
  Enable : EnablePort
  MATLAB Function4 : MATLAB Function  TreatAsAtomicUnit=on
  iterCount : Outport
  R_A : Outport  Port=2
  T : Outport  Port=3
  dev_A : Outport  Port=4
  ScanTime : Outport  Port=5
  wires:
  data_set/1 -> MATLAB Function4/1(data_set)
  model_set/1 -> MATLAB Function4/2(model_set)
  N_d/1 -> MATLAB Function4/3(N_d)
  N_m/1 -> MATLAB Function4/4(N_m)
  B_init/1 -> MATLAB Function4/5(B_init)
  maxIter/1 -> MATLAB Function4/6(maxIter)
  MATLAB Function4/1(iterCount) -> iterCount/1
  MATLAB Function4/2(R_A) -> R_A/1
  MATLAB Function4/3(T) -> T/1
  SigmaMult/1 -> MATLAB Function4/7(sigmaMult)
  alphaIn/1 -> MATLAB Function4/8(alphaIn)
  scanTime/1 -> MATLAB Function4/9(scanTime)
  MATLAB Function4/5(ScanTime) -> ScanTime/1
  MATLAB Function4/4(dev_A) -> dev_A/1

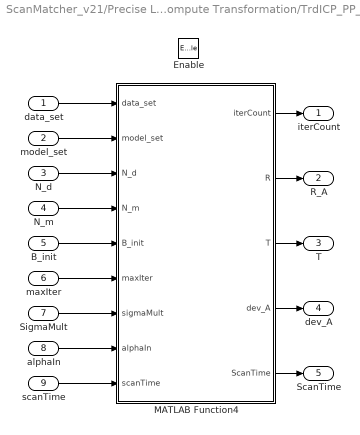
== system ScanMatcher_v21/Precise Localization/Compute Transformation/TrdICP_PP_corr ==
  data_set : Inport
  model_set : Inport  Port=2
  N_d : Inport  Port=3
  N_m : Inport  Port=4
  B_init : Inport  Port=5
  maxIter : Inport  Port=6
  SigmaMult : Inport  Port=7
  alphaIn : Inport  Port=8
  scanTime : Inport  Port=9
  Enable : EnablePort
  MATLAB Function4 : MATLAB Function  TreatAsAtomicUnit=on
  iterCount : Outport
  R_A : Outport  Port=2
  T : Outport  Port=3
  dev_A : Outport  Port=4
  ScanTime : Outport  Port=5
  wires:
  data_set/1 -> MATLAB Function4/1(data_set)
  model_set/1 -> MATLAB Function4/2(model_set)
  N_d/1 -> MATLAB Function4/3(N_d)
  N_m/1 -> MATLAB Function4/4(N_m)
  B_init/1 -> MATLAB Function4/5(B_init)
  maxIter/1 -> MATLAB Function4/6(maxIter)
  MATLAB Function4/1(iterCount) -> iterCount/1
  MATLAB Function4/2(R) -> R_A/1
  MATLAB Function4/3(T) -> T/1
  SigmaMult/1 -> MATLAB Function4/7(sigmaMult)
  alphaIn/1 -> MATLAB Function4/8(alphaIn)
  scanTime/1 -> MATLAB Function4/9(scanTime)
  MATLAB Function4/5(ScanTime) -> ScanTime/1
  MATLAB Function4/4(dev_A) -> dev_A/1

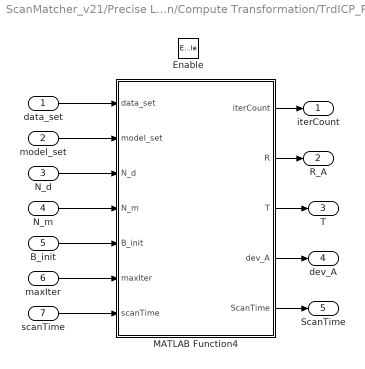
== system ScanMatcher_v21/Precise Localization/Compute Transformation/TrdICP_PP_ls ==
  data_set : Inport
  model_set : Inport  Port=2
  N_d : Inport  Port=3
  N_m : Inport  Port=4
  B_init : Inport  Port=5
  maxIter : Inport  Port=6
  scanTime : Inport  Port=7
  Enable : EnablePort
  MATLAB Function4 : MATLAB Function  TreatAsAtomicUnit=on
  iterCount : Outport
  R_A : Outport  Port=2
  T : Outport  Port=3
  dev_A : Outport  Port=4
  ScanTime : Outport  Port=5
  wires:
  data_set/1 -> MATLAB Function4/1(data_set)
  model_set/1 -> MATLAB Function4/2(model_set)
  N_d/1 -> MATLAB Function4/3(N_d)
  N_m/1 -> MATLAB Function4/4(N_m)
  B_init/1 -> MATLAB Function4/5(B_init)
  maxIter/1 -> MATLAB Function4/6(maxIter)
  MATLAB Function4/1(iterCount) -> iterCount/1
  MATLAB Function4/2(R) -> R_A/1
  MATLAB Function4/3(T) -> T/1
  scanTime/1 -> MATLAB Function4/7(scanTime)
  MATLAB Function4/5(ScanTime) -> ScanTime/1
  MATLAB Function4/4(dev_A) -> dev_A/1

== matlab function ScanMatcher_v21/Precise Localization/Compute Transformation/AfICP_PP_corr/MATLAB Function4 ==
  data: data_set input size=[2,2000]; model_set input size=[2,2000]; N_d input size=1 [..2000]; N_m input size=1 [..2000]; iterCount output; R_A output; B_init input; maxIter input; T output; dev_A output; sigmaMult input; alphaIn input; scanTime input; ScanTime output
function [iterCount,R_A,T,dev_A,ScanTime] = FindTransform(data_set,model_set,N_d,N_m,B_init,maxIter,sigmaMult,alphaIn,scanTime)
%%%%%%%%%%%%%%%%%%%%%%%%%%%%%%%%%%%%%%%%%%%%%%%%%%%%%%%%%%%%%%%%%%%%%%%%%%%
%%%%%%%%%%%%%%%% Affine ICP, Correntropy, Point to Point %%%%%%%%%%%%%%%%%%%
%%%%%%%%%%%%%%%%%%%%%%%%%%%%%%%%%%%%%%%%%%%%%%%%%%%%%%%%%%%%%%%%%%%%%%%%%%%
% Author  : Abdurrahman YILMAZ
% Date    : 15.09.2021
% Version : v01
% Notes   : ICP based 2D pose estimator. It takes model and data 
% clouds in 2D, target pose and initial pose information, and estimates 
% current pose
%%%%%%%%%%%%%%%%%%%%%%%%%%%%%%%%%%%%%%%%%%%%%%%%%%%%%%%%%%%%%%%%%%%%%%%%%%
    
    if isempty(maxIter) || isnan(maxIter) || isinf(maxIter) || maxIter <= 0 || maxIter >= 500
        maxNumIter = int32(100); % default value
    else
        maxNumIter = maxIter; % taken as ros paramter
    end
    
    if isempty(sigmaMult) || isnan(sigmaMult) || isinf(sigmaMult) || sigmaMult <= 0 || sigmaMult >= 100
        sigmaMultiplier = double(1); % default value
    else
        sigmaMultiplier = sigmaMult; % taken as ros paramter
    end
    
    if isempty(alphaIn) || isnan(alphaIn) || isinf(alphaIn) || alphaIn <= 0 || alphaIn >= 1
        alpha = double(0.8); % default value
    else
        alpha = alphaIn; % taken as ros paramter
    end
    
    sigma = 1;
    sigma_km1 = 0.1;
    B_km1 = B_init;
    B_k = B_init;
    count_stop_iter = 0;
    iterCount = int16(0);
    
    model_in = model_set';
    data_in = data_set';
    
%     N_model = nnz(~isnan(model_in))/2;
%     N_data = nnz(~isnan(data_in))/2;
    
    N_model = N_m;
    N_data = N_d;
    model= model_in(1:N_model,:);
    M1 = model;
    M = [M1,ones(size(M1,1),1)];
    data = data_in(1:N_data,:);
    P1 = data;
    P = [P1,ones(size(P1,1),1)];
    g = zeros(1,size(P1,1));
        
%     p_k = zeros(N_data,1);
    mck = [zeros(size(P1,1),2),ones(size(P1,1),1)];
    
    for iter = 1:maxNumIter
        iterCount = iterCount + 1;
        mck = [zeros(size(P1,1),2),ones(size(P1,1),1)];
        Pbar = (B_km1*P')';
        Idx = knnsearch(M(:,1:2),Pbar(:,1:2),'k',1);
        mck(:,1:2) = M(Idx(:,1),1:2);
        
        DiffModelData = zeros(length(Pbar),1);
        for i=1:1:length(Pbar)
            DiffModelData(i,1)=sqrt((Pbar(i,1)-mck(i,1))^2+(Pbar(i,2)-mck(i,2))^2);
        end
%         if iter ==1
%             sigma = sigmaMultiplier*std(DiffModelData);
%         else
%             sigma = sigma_km1*alpha + sigmaMultiplier*(1 - alpha)*sqrt(3/kurtosis(DiffModelData)*std(DiffModelData)^2); % 3 is standard Gaussian curve kurtosis 
%         end
        if iter ==1
            sigma = sigmaMultiplier*median(DiffModelData)*alpha + (1 - alpha)*sqrt(3/kurtosis(DiffModelData)*std(DiffModelData)^2);
        else
            sigma = sigma_km1*alpha;
        end
        
        for i = 1:1:size(P1,1)
            g(i) = exp(-(norm(B_km1*P(i,:)'-mck(i,:)')^2/(2*sigma^2)));
        end
        
        D_g = diag(g);
        B_k = ((P'*D_g*P)^(-1)*P'*D_g*mck)';
        
        if abs(norm(B_km1(1:3,1:3))-norm(B_k(1:3,1:3))) < 0.0001
            count_stop_iter = count_stop_iter + 1;
            if count_stop_iter > 5
                break;
            end
        else
            count_stop_iter = 0;
        end
        
        B_km1 = B_k(1:3,1:3);
        sigma_km1 = sigma;
    end
        
    B_final = B_k(1:3,1:3);
    
    % Affine transformation A matrix and T vector
    A = B_final(1:2,1:2);
    T = B_final(1:2,3);
    
    S = real(sqrtm(A'*A));
    R_A = A*S^(-1);
    dev_A = norm(A - R_A);
    iterCount = int16(iterCount);
    ScanTime = scanTime;
    
%     for j = 1:1:N_data
%         p_k(j) = exp(-(norm(B_final*P(j,:)'-mck(j,:)')^2/(2*sigma^2)));
%     end
% 
%     sum_p_k = 0;
% 
%     for tt = 1:1:N_data
%         sum_p_k = sum_p_k + p_k(tt);
%     end
%     
%     sumForT = zeros(2,1);
%     for pp = 1:1:N_data
%         sumForT = sumForT + (mck(pp,1:2)'-R_A*P(pp,1:2)')*p_k(pp);
%     end
% 
%     T_upd = sumForT/sum_p_k;

== matlab function ScanMatcher_v21/Precise Localization/OdomArray/MATLAB Function2 ==
  data: quat_In input; theta output size=1 [..2000]
function theta = Quat2Euler(quat_In)

    eul = quat2eul(quat_In');
    eul_deg = rad2deg(eul);
    theta = eul_deg(1,1);
end

== matlab function ScanMatcher_v21/Precise Localization/MATLAB Function8 ==
  data: paramValue input; param output
function param = DecodeActiveLocalizator(paramValue)
    MethodId = paramValue;
    switch MethodId
        case 1 % TrdICP_PP_corr
            param = [1,0,0,0];
        case 2 % AfICP_PP_corr
            param = [0,1,0,0];
        case 3 % AfICP_PL_corr
            param = [0,0,1,0];
        case 4 % TrdICP_PP_ls
            param = [0,0,0,1];
        otherwise
            param = [0,0,0,1];
    end
end

== matlab function ScanMatcher_v21/Precise Localization/Compute Transformation/AfICP_PL_corr/MATLAB Function4 ==
  data: data_set input size=[2,2000]; model_set input size=[2,2000]; N_d input size=1 [..2000]; N_m input size=1 [..2000]; iterCount output; R_A output; B_init input; maxIter input; T output; dev_A output; sigmaMult input; alphaIn input; scanTime input; ScanTime output
function [iterCount,R_A,T,dev_A,ScanTime] = FindTransform(data_set,model_set,N_d,N_m,B_init,maxIter,sigmaMult,alphaIn,scanTime)
%%%%%%%%%%%%%%%%%%%%%%%%%%%%%%%%%%%%%%%%%%%%%%%%%%%%%%%%%%%%%%%%%%%%%%%%%%%
%%%%%%%%%%%%%%%% Affine ICP, Correntropy, Point to Line %%%%%%%%%%%%%%%%%%%
%%%%%%%%%%%%%%%%%%%%%%%%%%%%%%%%%%%%%%%%%%%%%%%%%%%%%%%%%%%%%%%%%%%%%%%%%%%
% Author  : Abdurrahman YILMAZ
% Date    : 01.09.2021
% Version : v01
% Notes   : ICP based 2D pose estimator. It takes model and data 
% clouds in 2D, target pose and initial pose information, and estimates 
% current pose
%%%%%%%%%%%%%%%%%%%%%%%%%%%%%%%%%%%%%%%%%%%%%%%%%%%%%%%%%%%%%%%%%%%%%%%%%%
    
    if isempty(maxIter) || isnan(maxIter) || isinf(maxIter) || maxIter <= 0 || maxIter >= 500
        maxNumIter = int32(100); % default value
    else
        maxNumIter = maxIter; % taken as ros paramter
    end
    
    if isempty(sigmaMult) || isnan(sigmaMult) || isinf(sigmaMult) || sigmaMult <= 0 || sigmaMult >= 100
        sigmaMultiplier = double(1); % default value
    else
        sigmaMultiplier = sigmaMult; % taken as ros paramter
    end
    
    if isempty(alphaIn) || isnan(alphaIn) || isinf(alphaIn) || alphaIn <= 0 || alphaIn >= 1
        alpha = double(0.8); % default value
    else
        alpha = alphaIn; % taken as ros paramter
    end
    
    sigma = 1;
    sigma_km1 = 0.1;
    B_km1 = B_init;
    B_k = B_init;
    count_stop_iter = 0;
    iterCount = int16(0);
    
    model_in = model_set';
    data_in = data_set';
    
%     N_model = nnz(~isnan(model_in))/2;
%     N_data = nnz(~isnan(data_in))/2;
    
    N_model = N_m;
    N_data = N_d;
    model= model_in(1:N_model,:);
    M1 = model;
    M = [M1,ones(size(M1,1),1)];
    data = data_in(1:N_data,:);
    P1 = data;
    P = [P1,ones(size(P1,1),1)];
    g = zeros(1,size(P1,1));
        
%     p_k = zeros(N_data,1);
    mck = [zeros(size(P1,1),2),ones(size(P1,1),1)];
    mck2 = [zeros(size(P1,1),2),ones(size(P1,1),1)];
    mck3 = [zeros(size(P1,1),2),ones(size(P1,1),1)];
    mck4 = [zeros(size(P1,1),2),ones(size(P1,1),1)];
    
    for iter = 1:maxNumIter
        iterCount = iterCount + 1;
        mck = [zeros(size(P1,1),2),ones(size(P1,1),1)];
        mck2 = [zeros(size(P1,1),2),ones(size(P1,1),1)];
        mck3 = [zeros(size(P1,1),2),ones(size(P1,1),1)];
        mck4 = [zeros(size(P1,1),2),ones(size(P1,1),1)];
        Pbar = (B_km1*P')';
        Idx = knnsearch(M(:,1:2),Pbar(:,1:2),'k',4);
        mck(:,1:2) = M(Idx(:,1),1:2);
        mck2(:,1:2) = M(Idx(:,2),1:2);
        mck3(:,1:2) = M(Idx(:,3),1:2);
        mck4(:,1:2) = M(Idx(:,4),1:2);
        
        DiffModelData = zeros(length(Pbar),1);
        for i=1:1:length(Pbar)
            DiffModelData(i,1)=sqrt((Pbar(i,1)-mck(i,1))^2+(Pbar(i,2)-mck(i,2))^2);
        end
%         if iter ==1
%             sigma = sigmaMultiplier*std(DiffModelData);
%         else
%             sigma = sigma_km1*alpha + sigmaMultiplier*(1 - alpha)*sqrt(3/kurtosis(DiffModelData)*std(DiffModelData)^2); % 3 is standard Gaussian curve kurtosis 
%         end
        if iter ==1
            sigma = sigmaMultiplier*median(DiffModelData)*alpha + (1 - alpha)*sqrt(3/kurtosis(DiffModelData)*std(DiffModelData)^2);
        else
            sigma = sigma_km1*alpha;
        end
        
        Q = zeros(6,6);
        G = zeros(1,6);
        
        for i = 1:1:N_data
            Ti = [P(i,1:2),zeros(1,2),1,0;zeros(1,2),P(i,1:2),0,1];
            fitted_line = polyfit([mck(i,1) mck2(i,1) mck3(i,1) mck4(i,1)],[mck(i,2) mck2(i,2) mck3(i,2) mck4(i,2)],1);
            y_fit = polyval(fitted_line,[mck(i,1) mck2(i,1) mck3(i,1) mck4(i,1)]);
            ni = [cosd(90),-sind(90);sind(90),cosd(90)]*([mck(i,1);y_fit(1,1)]-[mck2(i,1);y_fit(1,2)]);
            ni = ni/norm(ni);
            Ci = ni*ni';
            g(i) = exp(-(([ni;1]'*(B_km1*P(i,:)'-mck(i,:)'))^2/(2*sigma^2)));
            if ~isnan((Ti'*Ci*Ti)*g(i))
                Q = Q + (Ti'*Ci*Ti)*g(i);
                G = G + (mck(i,1:2)*Ci*Ti)*g(i);
            end
        end
        
        X = (G*Q^(-1))';
        if ~isnan(X)
            B_k = [X(1,1) X(2,1) X(5,1);...
                X(3,1) X(4,1) X(6,1);...
                0 0 1];
        end
        
        if abs(norm(B_km1(1:3,1:3))-norm(B_k(1:3,1:3))) < 0.0001
            count_stop_iter = count_stop_iter + 1;
            if count_stop_iter > 5
                break;
            end
        else
            count_stop_iter = 0;
        end
        
        B_km1 = B_k(1:3,1:3);
        sigma_km1 = sigma;
    end
        
    B_final = B_k(1:3,1:3);
    
    % Affine transformation A matrix and T vector
    A = B_final(1:2,1:2);
    T = B_final(1:2,3);
    
    S = real(sqrtm(A'*A));
    R_A = A*S^(-1);
    dev_A = norm(A - R_A);
    iterCount = int16(iterCount);
    ScanTime = scanTime;
    
%     for j = 1:1:N_data
%         p_k(j) = exp(-(norm(B_final*P(j,:)'-mck(j,:)')^2/(2*sigma^2)));
%     end
% 
%     sum_p_k = 0;
% 
%     for tt = 1:1:N_data
%         sum_p_k = sum_p_k + p_k(tt);
%     end
%     
%     sumForT = zeros(2,1);
%     for pp = 1:1:N_data
%         sumForT = sumForT + (mck(pp,1:2)'-R_A*P(pp,1:2)')*p_k(pp);
%     end
% 
%     T_upd = sumForT/sum_p_k;

== matlab function ScanMatcher_v21/Precise Localization/Compute Transformation/TrdICP_PP_ls/MATLAB Function4 ==
  data: data_set input size=[2,2000]; model_set input size=[2,2000]; N_d input size=1 [..2000]; N_m input size=1 [..2000]; iterCount output; R output; B_init input; maxIter input; T output; dev_A output; scanTime input; ScanTime output
function [iterCount,R,T,dev_A,ScanTime] = FindTransform(data_set,model_set,N_d,N_m,B_init,maxIter,scanTime)
%%%%%%%%%%%%%%%%%%%%%%%%%%%%%%%%%%%%%%%%%%%%%%%%%%%%%%%%%%%%%%%%%%%%%%%%%%%
%%%%%%%%%%%%%%%% Rigid ICP, Least-Square, Point to Point %%%%%%%%%%%%%%%%%%%
%%%%%%%%%%%%%%%%%%%%%%%%%%%%%%%%%%%%%%%%%%%%%%%%%%%%%%%%%%%%%%%%%%%%%%%%%%%
% Author  : Abdurrahman YILMAZ
% Date    : 15.09.2021
% Version : v01
% Notes   : ICP based 2D pose estimator. It takes model and data 
% clouds in 2D, target pose and initial pose information, and estimates 
% current pose
%%%%%%%%%%%%%%%%%%%%%%%%%%%%%%%%%%%%%%%%%%%%%%%%%%%%%%%%%%%%%%%%%%%%%%%%%%
    
    if isempty(maxIter) || isnan(maxIter) || isinf(maxIter) || maxIter <= 0 || maxIter >= 500
        maxNumIter = int32(100); % default value
    else
        maxNumIter = maxIter; % taken as ros paramter
    end

    B_km1 = B_init;
    B_k = B_init;
    count_stop_iter = 0;
    iterCount = int16(0);
    
    model_in = model_set';
    data_in = data_set';
    
%     N_model = nnz(~isnan(model_in))/2;
%     N_data = nnz(~isnan(data_in))/2;
    
    N_model = N_m;
    N_data = N_d;
    model= model_in(1:N_model,:);
    M1 = model;
    M = [M1,ones(size(M1,1),1)];
    data = data_in(1:N_data,:);
    P1 = data;
    P = [P1,ones(size(P1,1),1)];
        
%     p_k = zeros(N_data,1);
    mck = [];
    
    for iter = 1:maxNumIter
        iterCount = iterCount + 1;
        Pbar = (B_km1*P')';
        [Idx,Dist] = knnsearch(M(:,1:2),Pbar(:,1:2),'k',1);
        corr_points = [double(Idx),Dist,Pbar];
        corr_points = sortrows(corr_points,2);
                
        filterOutDist = median(Dist) + (median(Dist)-min(Dist));
        
        indexId = size(corr_points,1);
        
        for j = size(corr_points,1):-1:1
            if corr_points(j,2) <= filterOutDist
                indexId = j;
                break;
            end
        end
        
        Idx_filtered = corr_points(1:indexId,1);
        mck = [zeros(size(Idx_filtered,1),2),ones(size(Idx_filtered,1),1)];
        mck(:,1:2) = M(Idx_filtered,1:2);
        Pbar_trim = corr_points(1:indexId,3:4);
        
        number_of_model_points = size(mck,1);
        number_of_data_points = size(Pbar_trim,1);

        centroid_P = mean(Pbar_trim(:,1:2));
        centroid_M = mean(mck(:,1:2));
        
        H = (Pbar_trim(:,1:2)-repmat(centroid_P,number_of_data_points,1))'*(mck(:,1:2)-repmat(centroid_M,number_of_model_points,1));
        [U,~,V] = svd(H);
        R_k = V*U';
        
        if det(R_k) < 0
            V(:,2) = V(:,2)*(-1);
            R_k = V*U';
        end
        
        t_k = -R_k*centroid_P' + centroid_M';
        
        B_k = [R_k*B_km1(1:2,1:2),R_k*B_km1(1:2,3)+t_k;zeros(1,2),ones(1,1)];
                
        if abs(norm(B_km1(1:3,1:3))-norm(B_k(1:3,1:3))) < 0.0001
            count_stop_iter = count_stop_iter + 1;
            if count_stop_iter > 5
                break;
            end
        else
            count_stop_iter = 0;
        end
        
        B_km1 = B_k(1:3,1:3);
    end
        
    B_final = B_k(1:3,1:3);
    
    % Rigid transformation A matrix and T vector
    R = B_final(1:2,1:2);
    T = B_final(1:2,3);
    
    dev_A = 0;
    
    iterCount = int16(iterCount);
    ScanTime = scanTime;
